simulink model "untitled"  (R2024b)
settings: Solver=ode4  StartTime=0.0  StopTime=10  FixedStep=1/20  RelTol=1e-3
libraries: sldrtlib x1, ros2lib x1
settings Model: Creator=robot  LastModifiedBy=robot
settings OptimizationCC: DefaultParameterBehavior=Inlined  EnhancedBackFolding=on  PassReuseOutputArgsAs=Individual arguments  ZeroExternalMemoryAtStartup=off  ZeroInternalMemoryAtStartup=off  MaxStackSize=64  OptimizeBlockOrder=speed  DifferentSizesBufferReuse=on  OptimizationCustomize=off  EfficientTunableParamExpr=on
settings DebuggingCC: ParameterTunabilityLossMsg=error
settings HardwareCC: ProdBitPerLong=64  ProdHWDeviceType=Intel->x86-64 (Linux 64)
settings SFSimCC: MATLABDynamicMemAlloc=off
settings RTWCC: Description=Embedded Coder  SystemTargetFile=ert.tlc  HardwareBoard=Robot Operating System 2 (ROS 2)  TLCOptions="-aInlineSetEventsForThisBaseRateFcn=TLC_FALSE -aSuppressMultiTaskScheduler=TLC_FALSE  -aRateBasedStepFcn=0"  TemplateMakefile=ert_default_tmf  Toolchain=Colcon Tools  TargetLang=C++
settings CodeAppCC: ForceParamTrailComments=on  IgnoreCustomStorageClasses=off  OperatorAnnotations=on  SimulinkDataObjDesc=on  SFDataObjDesc=on  InsertBlockDesc=on
settings ERTTargetCC: CodeInterfacePackaging=C++ class  RootIOFormat=Structure reference

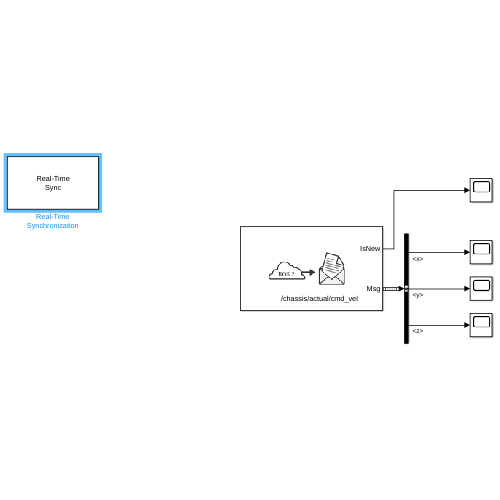
[thumbnail: Simulink's stored preview of the top-level diagram]
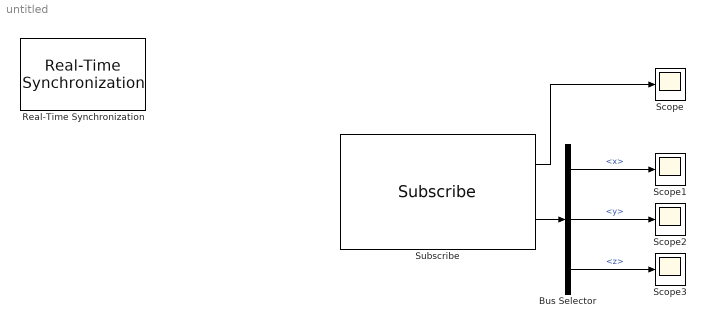
== system untitled ==
  Bus Selector : BusSelector  OutputSignals=twist.twist.linear.x,twist.twist.linear.y,twist.twist.angular.z
  Real-Time Synchronization : sldrtlib/Real-Time Synchronization  SampleTime=1/20  MaxMissedTicks=1000  ShowMissedTicks=off  YieldWhenWaiting=off
  Scope{,1..3} (4 alike) : Scope
  Subscribe : ros2lib/Subscribe  topicSource=Select from ROS network  topic=/chassis/actual/cmd_vel  messageType=geometry_msgs/TwistWithCovarianceStamped  sampleTime=-1  QOSHistory=Keep last  QOSDepth=1  QOSReliability=Reliable  QOSDurability=Volatile  QOSDeadline=Inf  QOSLifespan=Inf  QOSLiveliness=Automatic  QOSLeaseDuration=Inf  QOSAvoidROSNamespaceConventions=off
  wires:
  Bus Selector/1 -> Scope1/1  "<x>"
  Bus Selector/2 -> Scope2/1  "<y>"
  Bus Selector/3 -> Scope3/1  "<z>"
  Subscribe/2 -> Bus Selector/1
  Subscribe/1 -> Scope/1
